simulink model "ModelWithControllersOnly"  (R2021b)
settings: Solver=FixedStepAuto  StartTime=0.0  StopTime=10  RelTol=1e-3
model workspace (MAT data in the model file):
  firstWarning = 1
  originalScenarioChecksum = '114339432DE22364D47BB28FC96DC10C'
undefined symbols (not defined in the file): Acceleration, ActorID, AngularVelocity, DefaultGear, DEND_B, DEND_S, DEND_T, LF, LR, MAX_BRAKE, MAX_STEER, MAX_TORQUE, MCAR, MIN_BRAKE, MIN_STEER, MIN_TORQUE, NUMD_B, NUMD_S, NUMD_T, Pitch, Position, psi_o, R, Roll, RRdamp, session, sigbuilder_block, STEER_RATIO, Tdead, TrackWidth, ts, Vdead, Velocity, X_o, Y_o, Yaw
libraries: drivingvehiclecontroller x2, autolibshared x1, vehdynlibviscommon x1, vehdynlibsteering x1
settings Model: Creator=akshran  LastModifiedBy=Buckeye Autodrive
settings SolverCC: ConcurrentTasks=on  PositivePriorityOrder=on  AutoInsertRateTranBlk=on
settings DataIOCC: SignalLogging=off
settings OptimizationCC: BlockReduction=off  OptimizeBlockIOStorage=off
settings DebuggingCC: TasksWithSamePriorityMsg=none
settings HardwareCC: ProdBitPerLong=64  ProdLongLongMode=on  ProdHWDeviceType=Intel->x86-64 (Linux 64)
settings RTWCC: Description=Simulink Real-Time  SystemTargetFile=slrealtime.tlc  TemplateMakefile=slrealtime_default_tmf  Toolchain=Simulink Real-Time Toolchain  BuildConfiguration=Faster Runs  CodeExecutionProfiling=on  TargetLang=C++

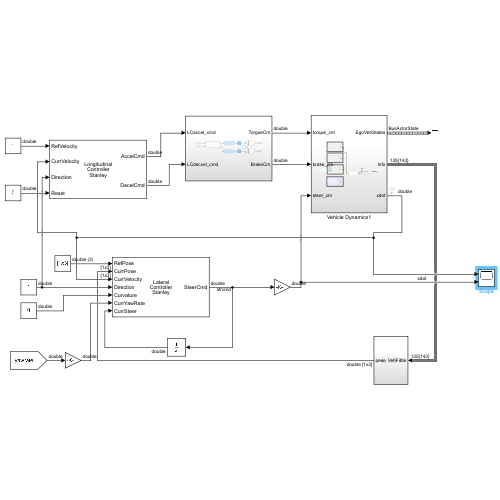
[thumbnail: Simulink's stored preview of the top-level diagram]
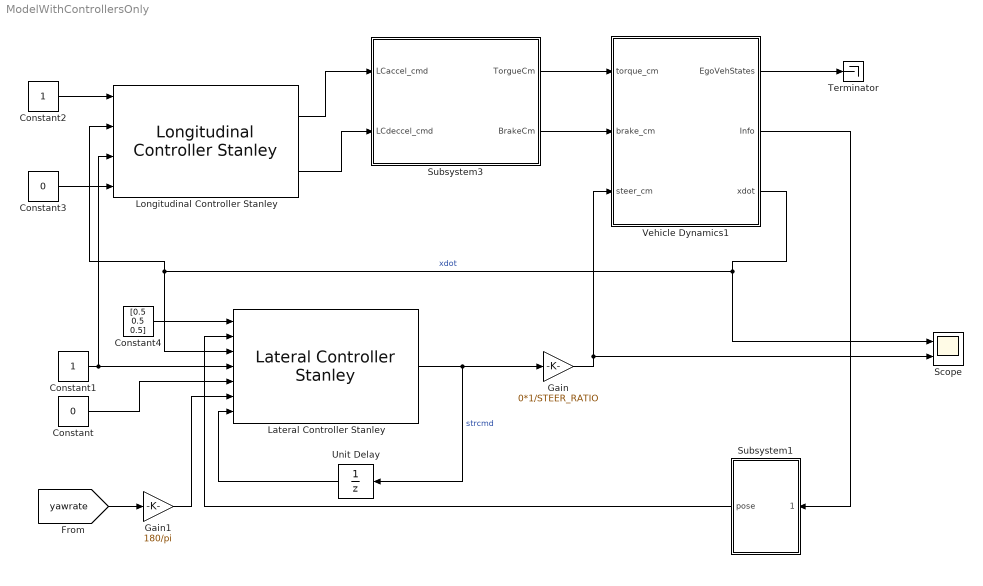
== system ModelWithControllersOnly ==
  Constant : Constant  Value=0
  Constant1 : Constant
  Constant2 : Constant
  Constant3 : Constant  Value=0
  Constant4 : Constant  Value=[0.5 0.5 0.5]
  Gain : Gain  Gain=0*1/STEER_RATIO
  Gain1 : Gain  Gain=180/pi
  Lateral Controller Stanley : drivingvehiclecontroller/Lateral Controller Stanley  ModelType=Dynamic bicycle model  PositionGainF=2.5  PositionGainR=2.5  YawRateGain=0.2  DelayGain=0.2  VehicleMass=MCAR  Lf=LF  Lr=LR  TireStiffness=5e3  Wheelbase=3  MaxSteeringAngle=80
      settings: SourceProductBaseCode=DR
  Longitudinal Controller Stanley : drivingvehiclecontroller/Longitudinal Controller Stanley  Kp=10  Ki=2.5  SampleTime=0.05  MaxAcceleration=40  MaxDeceleration=40
      settings: SourceProductBaseCode=DR
  Scope : Scope  NumInputPorts=2
  Subsystem1 : Subsystem
  Subsystem3 : Subsystem
  Terminator : Terminator
  Unit Delay : UnitDelay  SampleTime=-1  HasFrameUpgradeWarning=on
  Vehicle Dynamics1 : Subsystem
  wires:
  Vehicle Dynamics1/2(Info) -> Subsystem1/1(VehFdbk)
  Constant3/1 -> Longitudinal Controller Stanley/4
  Vehicle Dynamics1/3(xdot) -> Longitudinal Controller Stanley/2, Lateral Controller Stanley/3, Scope/1  "xdot"
  [yawrate] -> Gain1/1
  Gain1/1 -> Lateral Controller Stanley/6
  Gain/1 -> Scope/2, Vehicle Dynamics1/3(steer_cm)
  Longitudinal Controller Stanley/1 -> Subsystem3/1(LCaccel_cmd)
  Longitudinal Controller Stanley/2 -> Subsystem3/2(LCdeccel_cmd)
  Subsystem3/1(TorgueCm) -> Vehicle Dynamics1/1(torque_cm)
  Subsystem3/2(BrakeCm) -> Vehicle Dynamics1/2(brake_cm)
  Subsystem1/1(pose) -> Lateral Controller Stanley/2
  Lateral Controller Stanley/1 -> Gain/1, Unit Delay/1  "strcmd"
  Constant2/1 -> Longitudinal Controller Stanley/1
  Unit Delay/1 -> Lateral Controller Stanley/7
  Vehicle Dynamics1/1(EgoVehStates) -> Terminator/1
  Constant/1 -> Lateral Controller Stanley/5
  Constant1/1 -> Longitudinal Controller Stanley/3, Lateral Controller Stanley/4
  Constant4/1 -> Lateral Controller Stanley/1

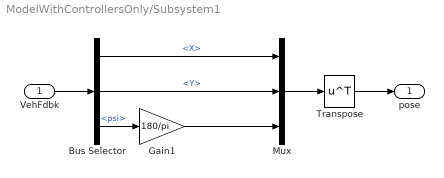
== system ModelWithControllersOnly/Subsystem1 ==
  VehFdbk : Inport
  Bus Selector : BusSelector  OutputSignals=InertFrm.Cg.Disp.X,InertFrm.Cg.Disp.Y,InertFrm.Cg.Ang.psi
  Gain1 : Gain  Gain=180/pi
  Mux : Mux  Inputs=3
  Transpose : Math  Operator=transpose  SignedPower=on  SaturateOnIntegerOverflow=on
  pose : Outport
  wires:
  Mux/1 -> Transpose/1
  VehFdbk/1 -> Bus Selector/1
  Gain1/1 -> Mux/3
  Transpose/1 -> pose/1
  Bus Selector/3 -> Gain1/1  "<psi>"
  Bus Selector/2 -> Mux/2  "<Y>"
  Bus Selector/1 -> Mux/1  "<X>"

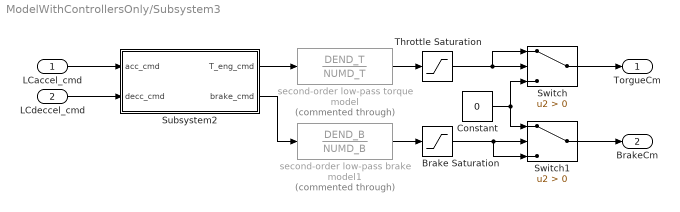
== system ModelWithControllersOnly/Subsystem3 ==
  LCaccel_cmd : Inport
  LCdeccel_cmd : Inport  Port=2
  Brake Saturation : Saturate  UpperLimit=MAX_BRAKE  LowerLimit=MIN_BRAKE
  Constant : Constant  Value=0
  Subsystem2 : Subsystem
  Switch : Switch  Criteria=u2 > Threshold
  Switch1 : Switch  Criteria=u2 > Threshold
  Throttle Saturation : Saturate  UpperLimit=MAX_TORQUE  LowerLimit=MIN_TORQUE
  second-order low-pass brake model1 : DiscreteTransferFcn  Commented=through  Numerator=DEND_B  Denominator=NUMD_B  SampleTime=ts
  second-order low-pass torque model : DiscreteTransferFcn  Commented=through  Numerator=DEND_T  Denominator=NUMD_T  SampleTime=ts
  TorgueCm : Outport
  BrakeCm : Outport  Port=2
  wires:
  Constant/1 -> Switch/3, Switch1/1
  Brake Saturation/1 -> Switch1/2, Switch1/3
  Throttle Saturation/1 -> Switch/2, Switch/1
  second-order low-pass brake model1/1 -> Brake Saturation/1
  second-order low-pass torque model/1 -> Throttle Saturation/1
  Subsystem2/2(brake_cmd) -> second-order low-pass brake model1/1
  Subsystem2/1(T_eng_cmd) -> second-order low-pass torque model/1
  Switch/1 -> TorgueCm/1
  Switch1/1 -> BrakeCm/1
  LCaccel_cmd/1 -> Subsystem2/1(acc_cmd)
  LCdeccel_cmd/1 -> Subsystem2/2(decc_cmd)

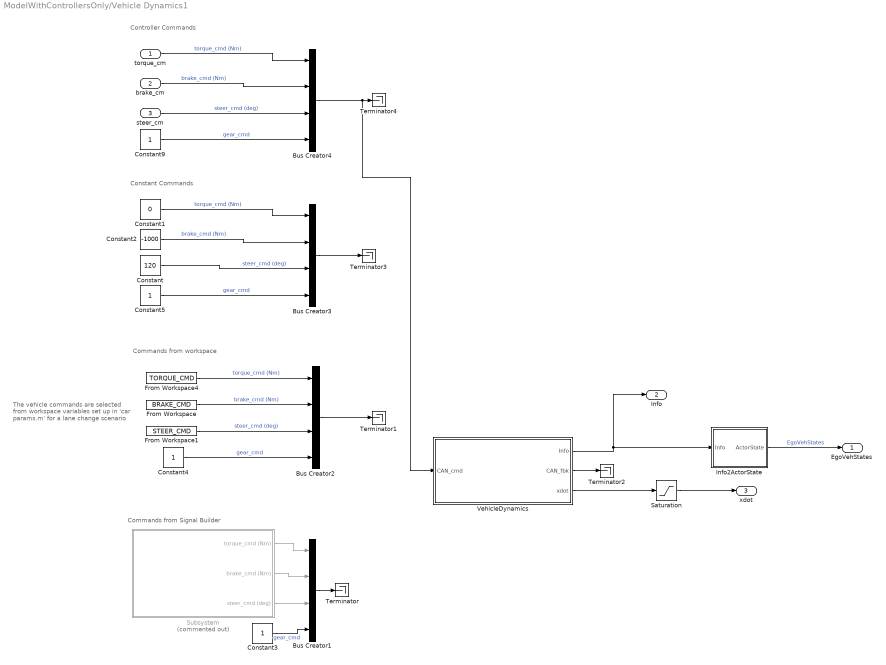
== system ModelWithControllersOnly/Vehicle Dynamics1 ==
  note: Constant Commands
  note: Commands from workspace
  note: Commands from Signal Builder
  note: The vehicle commands are selected from workspace variables set up in 'car params.m' for a lane change scenario
  note: Controller Commands
  torque_cm : Inport
  brake_cm : Inport  Port=2
  steer_cm : Inport  Port=3
  Bus Creator{1..4} (4 alike) : BusCreator  Inputs=4
  Constant : Constant  Value=120
  Constant1 : Constant  Value=0
  Constant2 : Constant  Value=-1000
  Constant{3..5,9} (4 alike) : Constant
  From Workspace : FromWorkspace  VariableName=BRAKE_CMD  SampleTime=ts
  From Workspace1 : FromWorkspace  VariableName=STEER_CMD  SampleTime=ts
  From Workspace4 : FromWorkspace  VariableName=TORQUE_CMD  SampleTime=ts
  Info2ActorState : Subsystem
  Saturation : Saturate  UpperLimit=inf  LowerLimit=0.001
  Subsystem : Subsystem  Commented=on
  Terminator{,1..4} (5 alike) : Terminator
  VehicleDynamics : Subsystem  mask{InitPosition=[X_o Y_o 0], InitSpeed=0, InitYaw=psi_o}
      mask prompts: InitPosition "Initial Position (m)"; InitSpeed "Initial Speed (m/s)"; InitYaw "Init Yaw (rad)"
  EgoVehStates : Outport
  Info : Outport  Port=2
  xdot : Outport  Port=3
  wires:
  Bus Creator2/1 -> Terminator1/1
  VehicleDynamics/2(CAN_fbk) -> Terminator2/1
  VehicleDynamics/1(Info) -> Info/1, Info2ActorState/1(Info)
  Constant/1 -> Bus Creator3/3  "steer_cmd (deg)"
  Info2ActorState/1(ActorState) -> EgoVehStates/1  "EgoVehStates"
  Constant1/1 -> Bus Creator3/1  "torque_cmd (Nm)"
  Constant2/1 -> Bus Creator3/2  "brake_cmd (Nm)"
  VehicleDynamics/3(xdot) -> Saturation/1
  Subsystem/1(torque_cmd (Nm)) -> Bus Creator1/1
  Subsystem/2(brake_cmd (Nm)) -> Bus Creator1/2
  Subsystem/3(steer_cmd (deg)) -> Bus Creator1/3
  Constant3/1 -> Bus Creator1/4  "gear_cmd"
  Constant4/1 -> Bus Creator2/4  "gear_cmd"
  From Workspace/1 -> Bus Creator2/2  "brake_cmd (Nm)"
  From Workspace1/1 -> Bus Creator2/3  "steer_cmd (deg)"
  From Workspace4/1 -> Bus Creator2/1  "torque_cmd (Nm)"
  Constant5/1 -> Bus Creator3/4  "gear_cmd"
  Bus Creator1/1 -> Terminator/1
  brake_cm/1 -> Bus Creator4/2  "brake_cmd (Nm)"
  Constant9/1 -> Bus Creator4/4  "gear_cmd"
  torque_cm/1 -> Bus Creator4/1  "torque_cmd (Nm)"
  steer_cm/1 -> Bus Creator4/3  "steer_cmd (deg)"
  Bus Creator3/1 -> Terminator3/1
  Bus Creator4/1 -> VehicleDynamics/1(CAN_cmd), Terminator4/1
  Saturation/1 -> xdot/1

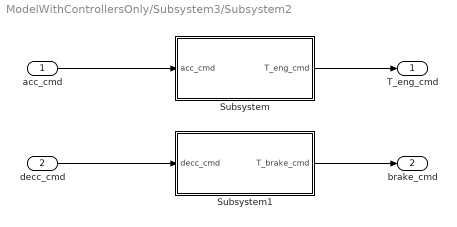
== system ModelWithControllersOnly/Subsystem3/Subsystem2 ==
  acc_cmd : Inport
  decc_cmd : Inport  Port=2
  Subsystem : Subsystem
  Subsystem1 : Subsystem
  T_eng_cmd : Outport
  brake_cmd : Outport  Port=2
  wires:
  acc_cmd/1 -> Subsystem/1(acc_cmd)
  Subsystem/1(T_eng_cmd) -> T_eng_cmd/1
  decc_cmd/1 -> Subsystem1/1(decc_cmd)
  Subsystem1/1(T_brake_cmd) -> brake_cmd/1

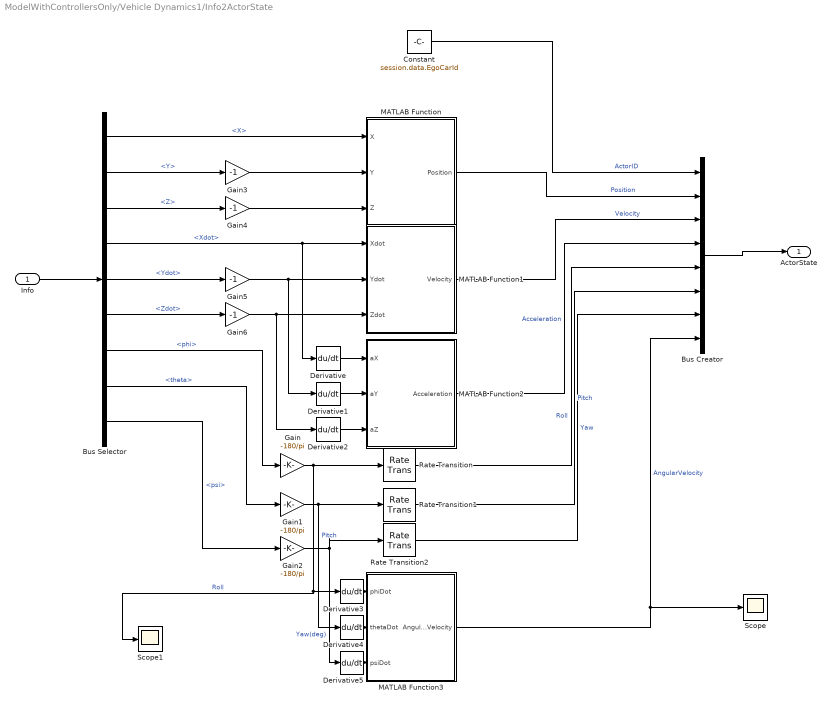
== system ModelWithControllersOnly/Vehicle Dynamics1/Info2ActorState ==
  Info : Inport
  Bus Creator : BusCreator  Inputs=ActorID,Position,Velocity,Acceleration,Roll,Pitch,Yaw,AngularVelocity  OutDataTypeStr=Bus: BusActorState  NonVirtualBus=on
  Bus Selector : BusSelector  OutputSignals=InertFrm.Cg.Disp.X,InertFrm.Cg.Disp.Y,InertFrm.Cg.Disp.Z,InertFrm.Cg.Vel.Xdot,InertFrm.Cg.Vel.Ydot,InertFrm.Cg.Vel.Zdot,InertFrm.Cg.Ang.phi,InertFrm.Cg.Ang.theta,InertFrm.Cg.Ang.psi
  Constant : Constant  Value=session.data.EgoCarId  SampleTime=0.05
  Derivative{,1..5} (6 alike) : Derivative
  Gain : Gain  Gain=-180/pi
  Gain1 : Gain  Gain=-180/pi
  Gain2 : Gain  Gain=-180/pi
  Gain{3..6} (4 alike) : Gain  Gain=-1
  MATLAB Function : MATLAB Function  TreatAsAtomicUnit=on  SystemSampleTime=0.05
  MATLAB Function1 : MATLAB Function  TreatAsAtomicUnit=on  SystemSampleTime=0.05
  MATLAB Function2 : MATLAB Function  TreatAsAtomicUnit=on  SystemSampleTime=0.05
  MATLAB Function3 : MATLAB Function  TreatAsAtomicUnit=on  SystemSampleTime=0.05
  Rate Transition : RateTransition  OutPortSampleTime=0.05
  Rate Transition1 : RateTransition  OutPortSampleTime=0.05
  Rate Transition2 : RateTransition  OutPortSampleTime=0.05
  Scope : Scope
  Scope1 : Scope
  ActorState : Outport
  wires:
  Gain/1 -> Scope1/1, Derivative3/1, Rate Transition/1  "Roll"
  Derivative4/1 -> MATLAB Function3/2(thetaDot)
  Bus Selector/2 -> Gain3/1  "<Y>"
  Bus Selector/4 -> Derivative/1, MATLAB Function1/1(Xdot)  "<Xdot>"
  MATLAB Function1/1(Velocity) -> Bus Creator/3  "Velocity"
  MATLAB Function/1(Position) -> Bus Creator/2  "Position"
  Derivative1/1 -> MATLAB Function2/2(aY)
  Bus Selector/5 -> Gain5/1  "<Ydot>"
  Bus Selector/1 -> MATLAB Function/1(X)  "<X>"
  Bus Selector/9 -> Gain2/1  "<psi>"
  Gain2/1 -> Rate Transition2/1, Derivative5/1  "Yaw(deg)"
  Derivative5/1 -> MATLAB Function3/3(psiDot)
  Bus Selector/7 -> Gain/1  "<phi>"
  MATLAB Function2/1(Acceleration) -> Bus Creator/4  "Acceleration"
  Derivative3/1 -> MATLAB Function3/1(phiDot)
  Gain1/1 -> Derivative4/1, Rate Transition1/1  "Pitch"
  Bus Selector/6 -> Gain6/1  "<Zdot>"
  Bus Selector/8 -> Gain1/1  "<theta>"
  MATLAB Function3/1(AngularVelocity) -> Bus Creator/8, Scope/1  "AngularVelocity"
  Bus Selector/3 -> Gain4/1  "<Z>"
  Derivative2/1 -> MATLAB Function2/3(aZ)
  Derivative/1 -> MATLAB Function2/1(aX)
  Info/1 -> Bus Selector/1
  Constant/1 -> Bus Creator/1  "ActorID"
  Bus Creator/1 -> ActorState/1
  Rate Transition/1 -> Bus Creator/5  "Roll"
  Rate Transition1/1 -> Bus Creator/6  "Pitch"
  Rate Transition2/1 -> Bus Creator/7  "Yaw"
  Gain3/1 -> MATLAB Function/2(Y)
  Gain4/1 -> MATLAB Function/3(Z)
  Gain5/1 -> Derivative1/1, MATLAB Function1/2(Ydot)
  Gain6/1 -> Derivative2/1, MATLAB Function1/3(Zdot)

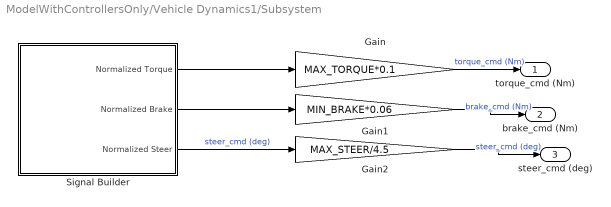
== system ModelWithControllersOnly/Vehicle Dynamics1/Subsystem ==
  Gain : Gain  Gain=MAX_TORQUE*0.1
  Gain1 : Gain  Gain=MIN_BRAKE*0.06
  Gain2 : Gain  Gain=MAX_STEER/4.5
  Signal Builder : Subsystem  Tag=STV Subsys  LoadFcn=sigbuilder_block('load');  StartFcn=sigbuilder_block('start');  StopFcn=sigbuilder_block('stop');  ClipboardFcn=sigbuilder_block('clipboard');  mask(Sigbuilder block){tuvar=[0:10]}
      mask help: Simulink:masks:SigbuilderBlock_MD
      mask init:
      | if ~strcmp(get_param(bdroot(gcbh),'SimulationStatus'),'stopped') tuvar = sigbuilder_block('maskInit'); end
      settings: CopyFcn=sigbuilder_block('copy');  DeleteFcn=sigbuilder_block('delete');  ModelCloseFcn=sigbuilder_block('modelClose');  PreSaveFcn=sigbuilder_block('preSave');  PauseFcn=sigbuilder_block('pause');  ContinueFcn=sigbuilder_block('continue');  NameChangeFcn=sigbuilder_block('namechange');  OpenFcn=sigbuilder_block('open',[0 30 960 455.5 ]);  CloseFcn=sigbuilder_block('close');
      mask Display: plot(0, 0, 100, 100,[2, 2, 32, 32, 2], [68, 8, 8, 68, 68],[32, 2], [38, 38], [32, 19, 2],[53, 60, 44], [32, 17, 17, 2],[16, 16, 31, 31]);txt = getActiveGroup(gcbh);text(2, 100, txt,'verticalAlignment', 'top');
  torque_cmd (Nm) : Outport
  brake_cmd (Nm) : Outport  Port=2
  steer_cmd (deg) : Outport  Port=3
  wires:
  Gain2/1 -> steer_cmd (deg)/1  "steer_cmd (deg)"
  Signal Builder/1(Normalized Torque) -> Gain/1
  Signal Builder/2(Normalized Brake) -> Gain1/1
  Signal Builder/3(Normalized Steer) -> Gain2/1  "steer_cmd (deg)"
  Gain1/1 -> brake_cmd (Nm)/1  "brake_cmd (Nm)"
  Gain/1 -> torque_cmd (Nm)/1  "torque_cmd (Nm)"

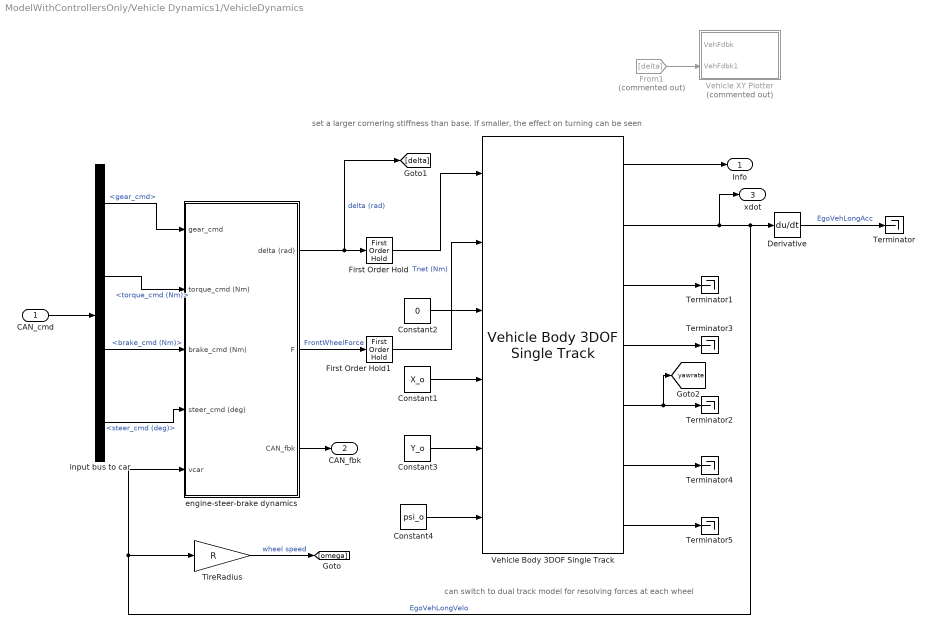
== system ModelWithControllersOnly/Vehicle Dynamics1/VehicleDynamics ==
  note: set a larger cornering stiffness than base. If smaller, the effect on turning can be seen
  note: can switch to dual track model for resolving forces at each wheel
  CAN_cmd : Inport
  Constant1 : Constant  Value=X_o
  Constant2 : Constant  Value=0
  Constant3 : Constant  Value=Y_o
  Constant4 : Constant  Value=psi_o
  Derivative : Derivative
  First Order Hold : FirstOrderHold  ErrorTolerance=inf
  First Order Hold1 : FirstOrderHold  ErrorTolerance=inf
  From1 : From  Commented=on  GotoTag=delta
  Terminator{,1..5} (6 alike) : Terminator
  TireRadius : Gain  Gain=R
  Vehicle Body 3DOF Single Track : autolibshared/Vehicle Body 3DOF Single Track  trackMode=Single (bicycle)  inputMode=External longitudinal forces  frontSteerMode=on  rearSteerMode=off  windMode=off  muMode=off  extFMode=off  extMMode=off  htchFMode=off  htchMMode=off  extXo=on  extpsio=on  extxdoto=off  extro=off  extYo=on  extTamb=off  extydoto=off  aMode=2  NF=2  NR=2  m=MCAR  a=LF  b=LR  h=0.35  dh=1  hh=0.2  X_o=InitPosition(1)  xdot_o=InitSpeed  CalphaMode=off  sigmaMode=on  d=0  hl=0  w=[1.4,1.4]  Cy_f=12e3*100  Cy_r=11e3*100  sigma_f=.1  sigma_r=.1  alpha_f_brk=[-.1 .1]  Cy_f_data=[-9e3 9e3]  alpha_r_brk=[-.1 .1]  Cy_r_data=[-9e3 9e3]  Y_o=-InitPosition(2)  ydot_o=0  Izz=2050  psi_o=-InitYaw/180*pi  r_o=0  Af=2  Cd=.3  Cl=.1  Cpm=.1  beta_w=[0:0.01:0.3]  Cs=[0:0.03:0.9]  Cym=[0:0.01:0.3]  Pabs=101325  Tair=273  g=9.81  mu=1  xdot_tol=.01  Fznom=5000  Fxtire_sat=7e4  Fytire_sat=7e4  longOff=0  latOff=0  vertOff=0  wrapAng=off
      settings: SourceProductBaseCode=PW,DR,MT,UV,VE
  Vehicle XY Plotter : Subsystem  Commented=on  mask(Vehicle XY Plotter){a=LF, b=LR, w=TrackWidth, bufferSize=1024, pltDT=.1}
      mask prompts: a "Distance to front axle from CG, a [m]:"; b "Distance to rear axle from CG, b [m]:"; w "Track width, w [m]:"; bufferSize "Path buffer sampe size, bufferSize []:"; pltDT "Plot update rate, pltDT [s]:"
      mask help: This block will display a MATLAB figure which indicates the vehicle path, current position and heading velocity.
      mask TypeOptions a: Vehicle XY Plotter/a
      mask TypeOptions b: Vehicle XY Plotter/b
      mask TypeOptions w: Vehicle XY Plotter/w
      mask TypeOptions bufferSize: Vehicle XY Plotter/bufferSize
  engine-steer-brake dynamics : Subsystem
  input bus to car : BusSelector  OutputSignals=gear_cmd,torque_cmd (Nm),brake_cmd (Nm),steer_cmd (deg)
  Info : Outport
  CAN_fbk : Outport  Port=2  VectorParamsAs1DForOutWhenUnconnected=off
  xdot : Outport  Port=3
  tag scope: yawrate=global
  wires:
  TireRadius/1 -> [omega]  "wheel speed"
  Vehicle Body 3DOF Single Track/1 -> Info/1
  From1/1 -> Vehicle XY Plotter/2(VehFdbk1)
  input bus to car/1 -> engine-steer-brake dynamics/1(gear_cmd)  "<gear_cmd>"
  input bus to car/3 -> engine-steer-brake dynamics/3(brake_cmd (Nm))  "<brake_cmd (Nm)>"
  engine-steer-brake dynamics/1(delta (rad)) -> [delta], First Order Hold/1  "delta (rad)"
  input bus to car/2 -> engine-steer-brake dynamics/2(torque_cmd (Nm))  "<torque_cmd (Nm)>"
  input bus to car/4 -> engine-steer-brake dynamics/4(steer_cmd (deg))  "<steer_cmd (deg)>"
  engine-steer-brake dynamics/3(CAN_fbk) -> CAN_fbk/1
  CAN_cmd/1 -> input bus to car/1
  Constant2/1 -> Vehicle Body 3DOF Single Track/3
  engine-steer-brake dynamics/2(F) -> First Order Hold1/1  "FrontWheelForce"
  First Order Hold/1 -> Vehicle Body 3DOF Single Track/1
  Vehicle Body 3DOF Single Track/2 -> xdot/1, engine-steer-brake dynamics/5(vcar), TireRadius/1, Derivative/1  "EgoVehLongVelo"
  Vehicle Body 3DOF Single Track/3 -> Terminator1/1
  Vehicle Body 3DOF Single Track/4 -> Terminator3/1
  Vehicle Body 3DOF Single Track/5 -> [yawrate], Terminator2/1
  Vehicle Body 3DOF Single Track/6 -> Terminator4/1
  Vehicle Body 3DOF Single Track/7 -> Terminator5/1
  Derivative/1 -> Terminator/1  "EgoVehLongAcc"
  First Order Hold1/1 -> Vehicle Body 3DOF Single Track/2  "Tnet (Nm)"
  Constant1/1 -> Vehicle Body 3DOF Single Track/4
  Constant3/1 -> Vehicle Body 3DOF Single Track/5
  Constant4/1 -> Vehicle Body 3DOF Single Track/6

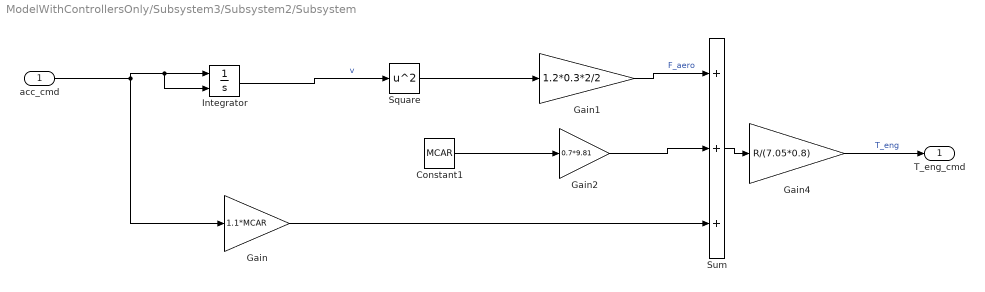
== system ModelWithControllersOnly/Subsystem3/Subsystem2/Subsystem ==
  acc_cmd : Inport
  Constant1 : Constant  Value=MCAR
  Gain : Gain  Gain=1.1*MCAR
  Gain1 : Gain  Gain=1.2*0.3*2/2
  Gain2 : Gain  Gain=0.7*9.81
  Gain4 : Gain  Gain=R/(7.05*0.8)
  Integrator : Integrator  ExternalReset=falling
  Square : Math  Operator=square  SaturateOnIntegerOverflow=on
  Sum : Sum  Inputs=+++
  T_eng_cmd : Outport
  wires:
  Constant1/1 -> Gain2/1
  Gain/1 -> Sum/3
  Sum/1 -> Gain4/1
  acc_cmd/1 -> Gain/1, Integrator/2, Integrator/1
  Gain2/1 -> Sum/2
  Gain1/1 -> Sum/1  "F_aero"
  Gain4/1 -> T_eng_cmd/1  "T_eng"
  Integrator/1 -> Square/1  "v"
  Square/1 -> Gain1/1

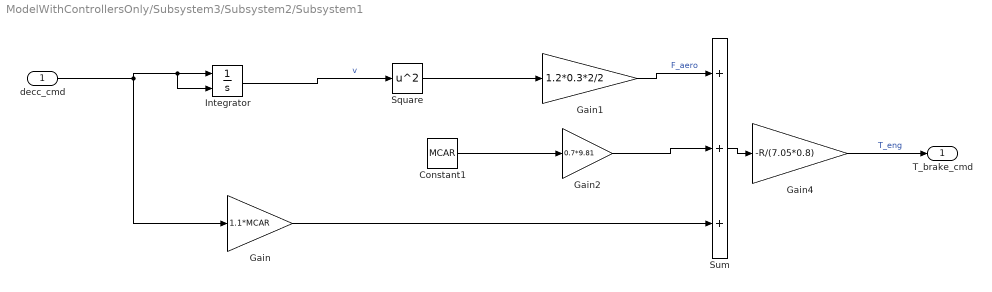
== system ModelWithControllersOnly/Subsystem3/Subsystem2/Subsystem1 ==
  decc_cmd : Inport
  Constant1 : Constant  Value=MCAR
  Gain : Gain  Gain=1.1*MCAR
  Gain1 : Gain  Gain=1.2*0.3*2/2
  Gain2 : Gain  Gain=0.7*9.81
  Gain4 : Gain  Gain=-R/(7.05*0.8)
  Integrator : Integrator  ExternalReset=falling
  Square : Math  Operator=square  SaturateOnIntegerOverflow=on
  Sum : Sum  Inputs=+++
  T_brake_cmd : Outport
  wires:
  Square/1 -> Gain1/1
  Integrator/1 -> Square/1  "v"
  Gain4/1 -> T_brake_cmd/1  "T_eng"
  Gain1/1 -> Sum/1  "F_aero"
  Gain2/1 -> Sum/2
  decc_cmd/1 -> Integrator/2, Integrator/1, Gain/1
  Sum/1 -> Gain4/1
  Gain/1 -> Sum/3
  Constant1/1 -> Gain2/1

== system ModelWithControllersOnly/Vehicle Dynamics1/Subsystem/Signal Builder ==
  Demux : Demux  Tag=STV Demux  Outputs=3
      settings: DisplayOption=none
  FromWs : FromWorkspace  Tag=STV FromWs  VariableName=tuvar
      SigBuilderData=|
      | common.afterFinalStr = 'Extrapolate'
      | common.sampleTime = 0
      | dataSet.timeRange = [0 3.5]
      | dataSet.name = 'DriveAndTurn'
      | sbobj.Groups.Name = 'DriveAndTurn'
      | sbobj.Groups.Signals(1).Name = 'Normalized Torque'
      | sbobj.Groups.Signals(1).XData = [0 1 1 2 2 3.5]
      | sbobj.Groups.Signals(1).YData = [1 1 0 0 1 1]
      | sbobj.Groups.Signals(2).Name = 'Normalized Brake'
      | sbobj.Groups.Signals(2).XData = [0 1 1 2 2 3.5]
      | sbobj.Groups.Signals(2).YData = [0 0 1 1 0 0]
      | sbobj.Groups.Signals(3).Name = 'Normalized Steer'
      | sbobj.Groups.Signals(3).XData = [0 0.5 0.6 1.02 1.02 2 2.5 3 3.5]
      | sbobj.Groups.Signals(3).YData = [-0.02 -0.02 -0.02 -0.3 -1.02 -0.92 -0.34 0.14 0.22]
      | sbobj.Groups.TimeRange = [0 3.5]
  Normalized Torque : Outport  Tag=STV Outport
  Normalized Brake : Outport  Tag=STV Outport  Port=2
  Normalized Steer : Outport  Tag=STV Outport  Port=3
  wires:
  FromWs/1 -> Demux/1
  Demux/1 -> Normalized Torque/1
  Demux/2 -> Normalized Brake/1
  Demux/3 -> Normalized Steer/1

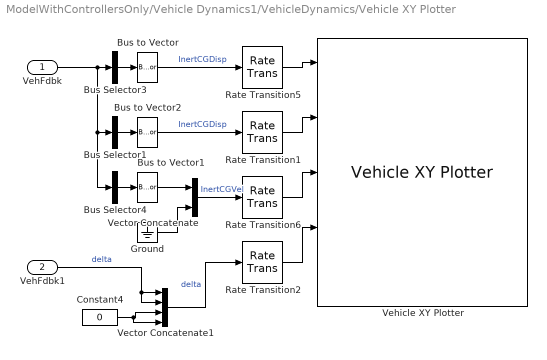
== system ModelWithControllersOnly/Vehicle Dynamics1/VehicleDynamics/Vehicle XY Plotter ==
  VehFdbk : Inport
  VehFdbk1 : Inport  Port=2
  Bus Selector1 : BusSelector  OutputSignals=InertFrm.Cg.Ang.phi,InertFrm.Cg.Ang.theta,InertFrm.Cg.Ang.psi  OutputAsBus=on
  Bus Selector3 : BusSelector  OutputSignals=InertFrm.Geom.Disp.X,InertFrm.Geom.Disp.Y,InertFrm.Geom.Disp.Z  OutputAsBus=on
  Bus Selector4 : BusSelector  OutputSignals=InertFrm.Cg.Vel.Xdot,InertFrm.Cg.Vel.Ydot  OutputAsBus=on
  Bus to Vector : BusToVector
  Bus to Vector1 : BusToVector
  Bus to Vector2 : BusToVector
  Constant4 : Constant  Value=0
  Ground : Ground
  Rate Transition{1..2,5..6} (4 alike) : RateTransition  OutPortSampleTime=pltDT
  Vector Concatenate : Concatenate
  Vector Concatenate1 : Concatenate  NumInputs=4
  Vehicle XY Plotter : vehdynlibviscommon/Vehicle XY Plotter  w=w  a=a  b=b  figBorder=2000  bufferSize=bufferSize  extStats=off  extTireF=off
      settings: SourceProductName=The database C:\Users\jrodgers\AppData\Roaming\MathWorks\MATLAB\R2018b\slblocks_master.db is locked, or a table in the database is locked. (database is locked)
  wires:
  Bus to Vector2/1 -> Rate Transition1/1  "InertCGDisp"
  Rate Transition5/1 -> Vehicle XY Plotter/1
  Bus Selector4/1 -> Bus to Vector1/1
  Rate Transition1/1 -> Vehicle XY Plotter/2
  Rate Transition6/1 -> Vehicle XY Plotter/3
  Vector Concatenate/1 -> Rate Transition6/1  "InertCGVel"
  Bus Selector1/1 -> Bus to Vector2/1
  Bus to Vector/1 -> Rate Transition5/1  "InertCGDisp"
  Bus Selector3/1 -> Bus to Vector/1
  Bus to Vector1/1 -> Vector Concatenate/1
  Ground/1 -> Vector Concatenate/2
  VehFdbk/1 -> Bus Selector1/1, Bus Selector4/1, Bus Selector3/1
  Rate Transition2/1 -> Vehicle XY Plotter/4
  Constant4/1 -> Vector Concatenate1/4, Vector Concatenate1/3
  VehFdbk1/1 -> Vector Concatenate1/2, Vector Concatenate1/1  "delta"
  Vector Concatenate1/1 -> Rate Transition2/1  "delta"

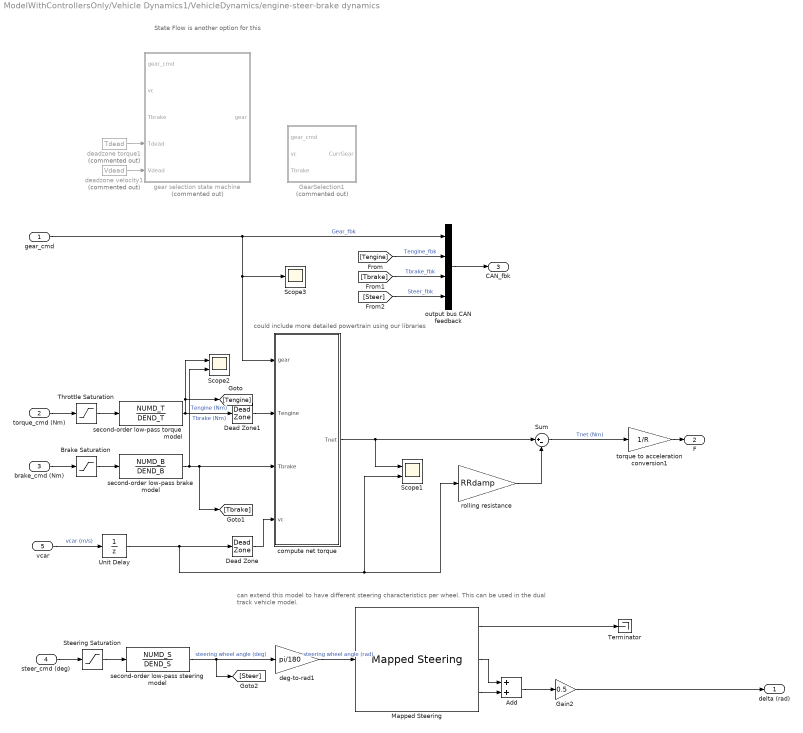
== system ModelWithControllersOnly/Vehicle Dynamics1/VehicleDynamics/engine-steer-brake dynamics ==
  note: State Flow is another option for this
  note: could include more detailed powertrain using our libraries
  note: can extend this model to have different steering characteristics per wheel. This can be used in the dual track vehicle model.
  gear_cmd : Inport
  torque_cmd (Nm) : Inport  Port=2
  brake_cmd (Nm) : Inport  Port=3
  steer_cmd (deg) : Inport  Port=4
  vcar : Inport  Port=5
  Add : Sum
  Brake Saturation : Saturate  UpperLimit=MAX_BRAKE  LowerLimit=MIN_BRAKE
  Dead Zone : DeadZone  LowerValue=-Vdead  UpperValue=Vdead  SaturateOnIntegerOverflow=on
  Dead Zone1 : DeadZone  LowerValue=-Tdead  UpperValue=Tdead  SaturateOnIntegerOverflow=on
  Gain2 : Gain  Gain=0.5
  GearSelection1 : Stateflow chart  Commented=on  TreatAsAtomicUnit=on  SystemSampleTime=ts
      settings: PortSchema="{\"entries\":[{\"content\":{\"sides\":[{\"content\":{\"connectorIds\":[\"In3\",\"In2\",\"In1\"]},\"type\":\"ConnectorPlacement.EquallySpacedRectSide\",\"uuid\":\"465e5722-891f-481b-b3b6-2b8339e8e743\"},{\"content\":{\"connectorIds\":[\"Out1\"],\"side\":\"RIGHT\"},\"type\":\"ConnectorPlacement.EquallySpacedRectSide\",\"uuid\":\"28ef13cd-41d9-4e2e-8cd9-9157abf573a9\"},{\"content\":{\"connectorIds\":[],\"side\":\"TOP\"},\"type\":\"ConnectorPlacement.EquallySpacedRectSide\",\"uuid\":\"44f19923-60ae-466f-ad2a-756f1033b52e\"},{\"content\":{\"connectorIds\":[],\"side\":\"HIDDEN\"},\"type\":\"ConnectorPlacement.EquallySpacedRectSide\",\"uuid\":\"d5a146f0-4328-42be-94e3-09f51634e7da\"}]},\"type\":\"ConnectorPlacement.EquallySpacedConnector\",\"uuid\":\"14e271af-3da2-4f7d-9688-fcc3c9792006\"}],\"packageUris\":[\"http://schema.mathworks.com/mf0/Connector/R2020b\"],\"version\":\"1.0\"}"
  Mapped Steering : vehdynlibsteering/Mapped Steering  SpdDpd=off  StrgAngBpts=[-1.5*pi 1.5*pi]  WhlLftTbl=[-1.5*pi 1.5*pi]*STEER_RATIO  WhlRghtTbl=[-1.5*pi 1.5*pi]*STEER_RATIO  VehSpdBpts=[-1 1]  SpdFctTbl=[1 1]  aMode=2
      settings: SourceProductBaseCode=VE
  Scope1 : Scope  NumInputPorts=2
  Scope2 : Scope  NumInputPorts=2
  Scope3 : Scope
  Steering Saturation : Saturate  UpperLimit=MAX_STEER  LowerLimit=MIN_STEER
  Sum : Sum  Inputs=|+-
  Terminator : Terminator
  Throttle Saturation : Saturate  UpperLimit=MAX_TORQUE  LowerLimit=MIN_TORQUE
  Unit Delay : UnitDelay  SampleTime=-1  HasFrameUpgradeWarning=on
  compute net torque : MATLAB Function  TreatAsAtomicUnit=on  SystemSampleTime=ts
  deadzone torque1 : Constant  Commented=on  Value=Tdead  SampleTime=ts
  deadzone velocity1 : Constant  Commented=on  Value=Vdead  SampleTime=ts
  deg-to-rad1 : Gain  Gain=pi/180
  gear selection state machine : MATLAB Function  Commented=on  TreatAsAtomicUnit=on  SystemSampleTime=ts
  output bus CAN feedback : BusCreator  Inputs=4
  rolling resistance : Gain  Gain=RRdamp
  second-order low-pass brake model : DiscreteTransferFcn  Numerator=NUMD_B  Denominator=DEND_B  SampleTime=ts
  second-order low-pass steering model : DiscreteTransferFcn  Numerator=NUMD_S  Denominator=DEND_S  SampleTime=ts
  second-order low-pass torque model : DiscreteTransferFcn  Numerator=NUMD_T  Denominator=DEND_T  SampleTime=ts
  torque to acceleration conversion1 : Gain  Gain=1/R
  delta (rad) : Outport  VectorParamsAs1DForOutWhenUnconnected=off
  F : Outport  Port=2  VectorParamsAs1DForOutWhenUnconnected=off
  CAN_fbk : Outport  Port=3  VectorParamsAs1DForOutWhenUnconnected=off
  wires:
  steer_cmd (deg)/1 -> Steering Saturation/1
  torque_cmd (Nm)/1 -> Throttle Saturation/1
  brake_cmd (Nm)/1 -> Brake Saturation/1
  second-order low-pass steering model/1 -> deg-to-rad1/1, [Steer]  "steering wheel angle (deg)"
  Throttle Saturation/1 -> second-order low-pass torque model/1
  Brake Saturation/1 -> second-order low-pass brake model/1
  Steering Saturation/1 -> second-order low-pass steering model/1
  vcar/1 -> Unit Delay/1  "vcar (m/s)"
  second-order low-pass brake model/1 -> [Tbrake], compute net torque/3(Tbrake), Scope2/2  "Tbrake (Nm)"
  second-order low-pass torque model/1 -> Dead Zone1/1, [Tengine], Scope2/1  "Tengine (Nm)"
  compute net torque/1(Tnet) -> Scope1/1, Sum/1
  rolling resistance/1 -> Sum/2
  deadzone velocity1/1 -> gear selection state machine/5(Vdead)
  deadzone torque1/1 -> gear selection state machine/4(Tdead)
  gear_cmd/1 -> output bus CAN feedback/1, Scope3/1, compute net torque/1(gear)  "Gear_fbk"
  output bus CAN feedback/1 -> CAN_fbk/1
  [Tengine] -> output bus CAN feedback/2  "Tengine_fbk"
  [Tbrake] -> output bus CAN feedback/3  "Tbrake_fbk"
  [Steer] -> output bus CAN feedback/4  "Steer_fbk"
  Mapped Steering/2 -> Add/1
  Mapped Steering/3 -> Add/2
  Add/1 -> Gain2/1
  torque to acceleration conversion1/1 -> F/1
  Mapped Steering/1 -> Terminator/1
  deg-to-rad1/1 -> Mapped Steering/1  "steering wheel angle (rad)"
  Sum/1 -> torque to acceleration conversion1/1  "Tnet (Nm)"
  Dead Zone/1 -> compute net torque/4(vc)
  Dead Zone1/1 -> compute net torque/2(Tengine)
  Unit Delay/1 -> Scope1/2, rolling resistance/1, Dead Zone/1
  Gain2/1 -> delta (rad)/1

== matlab function ModelWithControllersOnly/Vehicle Dynamics1/VehicleDynamics/engine-steer-brake dynamics/gear selection state machine ==
  data: gear output; gear_cmd input; vc input; Tbrake input; Tdead input; Vdead input
function gear = gear_change_FSM(gear_cmd,vc,Tbrake,Tdead,Vdead)

persistent GEAR

%  The vehicle gear can take on one of the following enumerated values:
%  -1 = REVERSE
%   0 = PARK
%   1 = DRIVE

%  --initialize the local persistent variables

if isempty(GEAR)
    %  --default gear at startup is PARK
    %  Note:  Change this to 1 if you want car to initialize in DRIVE
    GEAR = 0;
end


%  --evaluate the gear change finite state machine

switch GEAR
    case 0  % vehicle is in PARK
        if (gear_cmd == 1)
            %  --check to see if we can shift to DRIVE
            if ((abs(vc) <= Vdead) && (abs(Tbrake) > Tdead))
                %  --shift to DRIVE
                GEAR = 1;
            end
            
        elseif (gear_cmd == 2)
            %  --check to see if we can shift to REVERSE
            if ((abs(vc) <= Vdead) && (abs(Tbrake) > Tdead))
                %  --shift to REVERSE
                GEAR = 2;
            end
        end
        
    case 1  % vehicle is in DRIVE
        if (gear_cmd == 0)
            %  --check to see if we can shift to PARK
            if ((abs(vc) <= Vdead) && (abs(Tbrake) > Tdead))
                %  --shift to PARK
                GEAR = 0;
            end
            
        elseif (gear_cmd == 2)
            %  --check to see if we can shift to REVERSE
            if ((abs(vc) <= Vdead) && (abs(Tbrake) > Tdead))
                %  --shift to REVERSE
                GEAR = 2;
            end
        end
        
    case -1  % vehicle is in REVERSE
        if (gear_cmd == 0)
            %  --check to see if we can shift to PARK
            if ((abs(vc) <= Vdead) && (abs(Tbrake) > Tdead))
                %  --shift to PARK
                GEAR = 0;
            end
            
        elseif (gear_cmd == 1)
            %  --check to see if we can shift to DRIVE
            if ((abs(vc) <= Vdead) && (abs(Tbrake) > Tdead))
                %  --shift to DRIVE
                GEAR = 1;
            end
        end
        
    otherwise  %  --should never be here
        if (vc > Vdead)
            %  --moving forward, so must be in DRIVE
            GEAR = 1;
        elseif (vc < -Vdead)
            %  --moving backward, so must be in REVERSE
            GEAR = 2;
        else
            %  --vehicle stoppped, so must be in PARK
            GEAR = 0;
        end

end


%  --output the current actual gear setting

gear = GEAR;

return

== matlab function ModelWithControllersOnly/Vehicle Dynamics1/Info2ActorState/MATLAB Function ==
  data: X input; Position output; Y input; Z input
function Position = fcn(X, Y, Z)

Position = [X Y, Z];

== matlab function ModelWithControllersOnly/Vehicle Dynamics1/Info2ActorState/MATLAB Function1 ==
  data: Xdot input; Velocity output; Ydot input; Zdot input
function Velocity = fcn(Xdot, Ydot, Zdot)

Velocity = [Xdot Ydot, Zdot];

== matlab function ModelWithControllersOnly/Vehicle Dynamics1/Info2ActorState/MATLAB Function2 ==
  data: aX input; Acceleration output; aY input; aZ input
function Acceleration = fcn(aX, aY, aZ)

Acceleration = [aX aY, aZ];

== matlab function ModelWithControllersOnly/Vehicle Dynamics1/Info2ActorState/MATLAB Function3 ==
  data: phiDot input; AngularVelocity output; thetaDot input; psiDot input
function AngularVelocity = fcn(phiDot, thetaDot, psiDot)

AngularVelocity = [phiDot thetaDot, psiDot];

== stateflow chart ModelWithControllersOnly/Vehicle Dynamics1/VehicleDynamics/engine-steer-brake dynamics/GearSelection1 ==
  state Park
    CurrGear = 0;
  state Reverse
    CurrGear = -1;
  state drive
    CurrGear = 1;
  (default) -> (junction 12)
  (junction 12) -> Reverse [order 3] : [DefaultGear == -1]
  (junction 12) -> drive [order 2] : [DefaultGear == 1]
  (junction 12) -> Park [order 1] : [DefaultGear == 0]
  (junction 12) -> Park [order 4] : %fallback to park
  drive -> Park [order 2] : [gear_cmd == 0 && allowShift(vc,Tbrake)]
  Park -> Reverse [order 2] : [gear_cmd == -1 && allowShift(vc,Tbrake)]
  Park -> drive [order 1] : [gear_cmd == 1 && allowShift(vc,Tbrake)]
  Reverse -> Park [order 2] : [gear_cmd == 0 && allowShift(vc,Tbrake)]
  drive -> Reverse [order 1] : [gear_cmd == -1 && allowShift(vc,Tbrake)]
  Reverse -> drive [order 1] : [gear_cmd == 1 && allowShift(vc,Tbrake)]
  data: Tdead parameter; Vdead parameter; vel function_input; brakeT function_input; allow function_output; CurrGear output; Tbrake input; vc input; gear_cmd input; DefaultGear parameter
  function allow = allowShift(vel, brakeT):
    | function allow = allowShift(vel, brakeT)
    | allow = (abs(vel) <= Vdead) && (abs(brakeT)>Tdead);
    | end

== matlab function ModelWithControllersOnly/Vehicle Dynamics1/VehicleDynamics/engine-steer-brake dynamics/compute net torque ==
  data: gear input; Tnet output; Tengine input; Tbrake input; vc input
function Tnet  = net_torque(gear,Tengine,Tbrake,vc)

%  --set engine torque based on current gear selection

if (gear == 0)
    %  --vehicle is in PARK, so force engine torque to zero
    Tengine = 0;
end

Tnet = Tengine + Tbrake*tanh(5*vc);

end
